simulink model "IO424_Synchro_signal_gen"  (R2024b)
settings: Solver=FixedStepDiscrete  StartTime=0.0  StopTime=0.15  FixedStep=1e-6  RelTol=1e-3
settings Model: Creator=aleandro.vegni  LastModifiedBy=aleandro.vegni

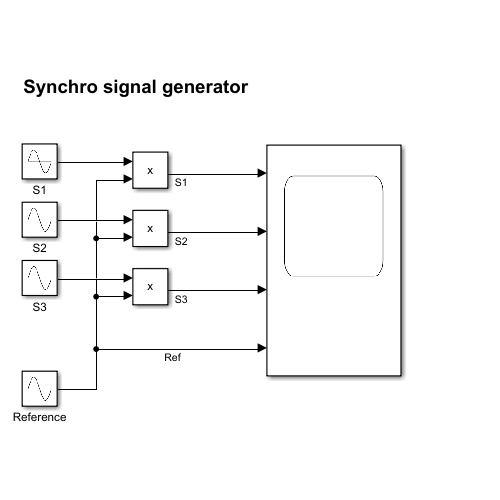
[thumbnail: Simulink's stored preview of the top-level diagram]
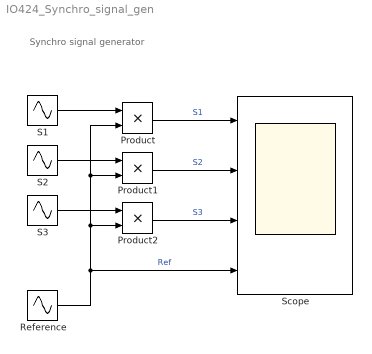
== system IO424_Synchro_signal_gen ==
  note: Synchro signal generator
  Product : Product
  Product1 : Product
  Product2 : Product
  Reference : Sin  Amplitude=4*sqrt(2)  Frequency=2*pi*1e3  SampleTime=0
  S1 : Sin  Amplitude=0.5  Frequency=2*pi*10  Phase=pi/2+(2*pi/3)  SampleTime=0
  S2 : Sin  Amplitude=0.5  Frequency=2*pi*10  Phase=pi/2  SampleTime=0
  S3 : Sin  Amplitude=0.5  Frequency=2*pi*10  Phase=pi/2+(4*pi/3)  SampleTime=0
  Scope : Scope  NumInputPorts=4
  wires:
  S1/1 -> Product/1
  S2/1 -> Product1/1
  S3/1 -> Product2/1
  Reference/1 -> Product2/2, Product/2, Product1/2, Scope/4  "Ref"
  Product/1 -> Scope/1  "S1"
  Product1/1 -> Scope/2  "S2"
  Product2/1 -> Scope/3  "S3"
